simulink model "untitled"  (R2023b)
settings: Solver=VariableStepAuto  StartTime=0.0  StopTime=4  RelTol=1e-6
settings Model: Creator=Rendszergazda  LastModifiedBy=Rendszergazda

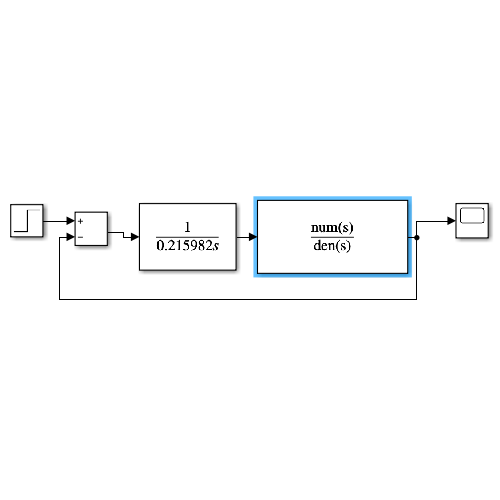
[thumbnail: Simulink's stored preview of the top-level diagram]
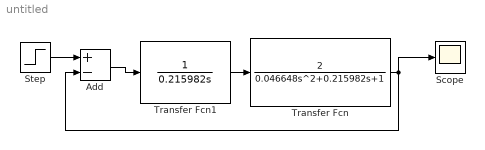
== system untitled ==
  Add : Sum  Inputs=+-
  Scope : Scope
  Step : Step  Time=0  SampleTime=0
  Transfer Fcn : TransferFcn  Numerator=[2]  Denominator=[0.046648 0.215982 1]
  Transfer Fcn1 : TransferFcn  Denominator=[0.215982 0]
  wires:
  Step/1 -> Add/1
  Add/1 -> Transfer Fcn1/1
  Transfer Fcn1/1 -> Transfer Fcn/1
  Transfer Fcn/1 -> Add/2, Scope/1
